simulink subsystem "TC_Target"  (R2021b)
settings: Solver=VariableStepAuto  StartTime=0.0  StopTime=10.0  RelTol=1e-3
undefined symbols (not defined in the file): afx_f, agx_f, BestSlipRate, gear_f, gear_r, Iwf, Load, mu_tire_F, Rwf, Rwr, SlipAngle
libraries: dspstat3 x2, simulink x2
settings Model: Creator=tsuyoshi  LastModifiedBy=tsuyoshi

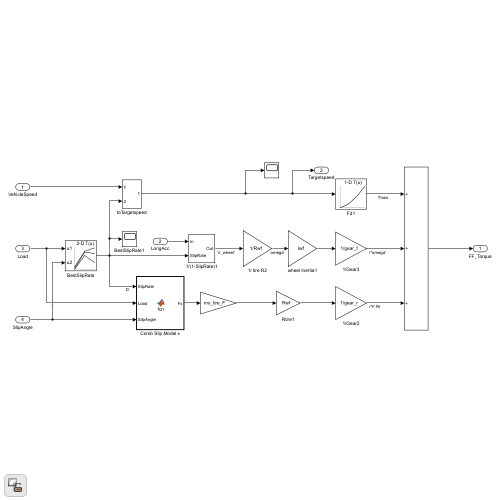
[thumbnail: Simulink's stored preview of the top-level diagram]
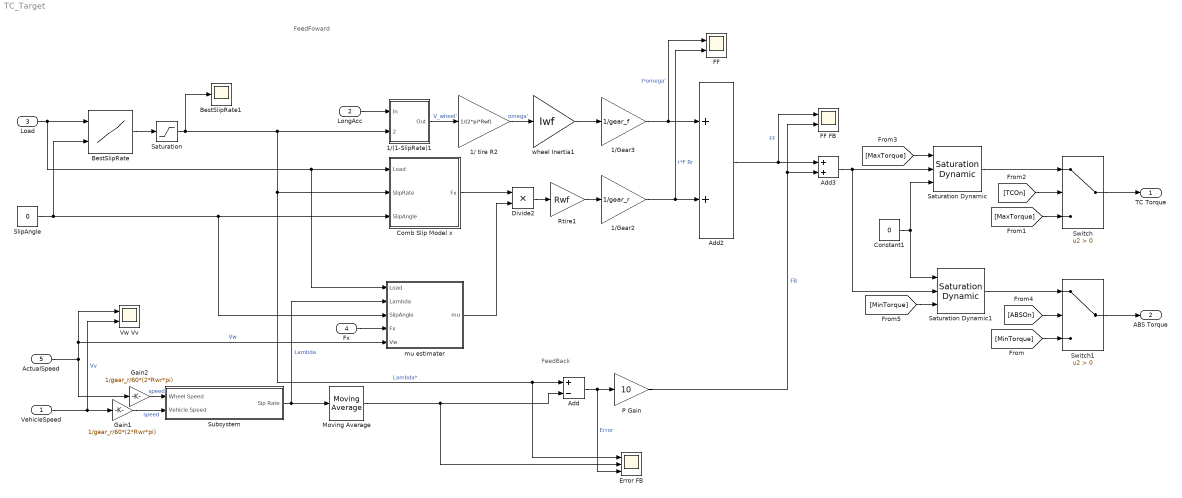
== system TC_Target ==
  note: FeedFoward
  note: FeedBack
  VehicleSpeed : Inport
  LongAcc : Inport  Port=2
  Load : Inport  Port=3
  Fx : Inport  Port=4
  ActualSpeed : Inport  Port=5
  1/ tire R2 : Gain  Gain=1/(2*pi*Rwf)
  1/(1-SlipRate)1 : Subsystem
  1/Gear2 : Gain  Gain=1/gear_r
  1/Gear3 : Gain  Gain=1/gear_f
  Add : Sum  Inputs=+-
  Add2 : Sum
  Add3 : Sum
  BestSlipRate : Lookup_n-D  BreakpointsForDimension1=Load  BreakpointsForDimension2=SlipAngle  Table=BestSlipRate  InternalRulePriority=Speed  RndMeth=Simplest  InputSameDT=on
      settings: InputPortMap=u0,u1
  BestSlipRate1 : Scope
  Comb Slip Model x : MATLAB Function  TreatAsAtomicUnit=on
  Constant1 : Constant  Value=0
  Divide2 : Product  Inputs=**
  Error FB : Scope  NumInputPorts=3
  FF : Scope  NumInputPorts=2
  FF FB : Scope  NumInputPorts=2
  Gain1 : Gain  Gain=1/gear_r/60*(2*Rwr*pi)
  Gain2 : Gain  Gain=1/gear_r/60*(2*Rwr*pi)
  Moving Average : dspstat3/Moving Average  Method=Sliding window  ForgettingFactorPort=off  SpecifyWindowLength=on  WindowLength=10  ForgettingFactor=0.9  SimulateUsing=Code generation
  P Gain : Gain  Gain=10
  Rtire1 : Gain  Gain=Rwf
  Saturation : Saturate  UpperLimit=0.3  LowerLimit=-0.3
  Saturation Dynamic : simulink/Discontinuities/Saturation Dynamic  OutMin=[]  OutMax=[]  OutDataTypeStr=Inherit: Same as second input  OutDataType=fixdt(1, 16)  OutScaling=2^-10  DoSatur=off
  Saturation Dynamic1 : simulink/Discontinuities/Saturation Dynamic  OutMin=[]  OutMax=[]  OutDataTypeStr=Inherit: Same as second input  OutDataType=fixdt(1, 16)  OutScaling=2^-10  DoSatur=off
  SlipAngle : Constant  Value=0
  Subsystem : Subsystem
  Switch : Switch  Criteria=u2 > Threshold
  Switch1 : Switch  Criteria=u2 > Threshold
  Vw Vv : Scope  NumInputPorts=2
  mu estimater : Subsystem
  wheel Inertia1 : Gain  Gain=Iwf
  TC Torque : Outport
  ABS Torque : Outport  Port=2
  wires:
  mu estimater/1(mu) -> Divide2/2
  Fx/1 -> mu estimater/4(Fx)
  Comb Slip Model x/1(Fx) -> Divide2/1
  Divide2/1 -> Rtire1/1
  Subsystem/1(Sip Rate) -> mu estimater/2(Lambda), Moving Average/1  "Lambda"
  Switch1/1 -> ABS Torque/1
  [MinTorque] -> Saturation Dynamic1/3
  Saturation Dynamic1/1 -> Switch1/1
  [ABSOn] -> Switch1/2
  [MinTorque] -> Switch1/3
  [MaxTorque] -> Saturation Dynamic/1
  Constant1/1 -> Saturation Dynamic/3, Saturation Dynamic1/1
  Switch/1 -> TC Torque/1
  Saturation Dynamic/1 -> Switch/1
  [TCOn] -> Switch/2
  Add3/1 -> Saturation Dynamic1/2, Saturation Dynamic/2
  [MaxTorque] -> Switch/3
  P Gain/1 -> Add3/2, FF FB/2  "FB"
  Add2/1 -> FF FB/1, Add3/1  "FF"
  Add/1 -> Error FB/3, P Gain/1  "Error"
  VehicleSpeed/1 -> Vw Vv/2, Gain1/1  "Vv"
  ActualSpeed/1 -> mu estimater/5(Vw), Vw Vv/1, Gain2/1  "Vw"
  BestSlipRate/1 -> Saturation/1
  SlipAngle/1 -> BestSlipRate/2, mu estimater/3(SlipAngle), Comb Slip Model x/3(SlipAngle)
  LongAcc/1 -> 1/(1-SlipRate)1/1(In)
  1/Gear3/1 -> FF/1, Add2/1  "I*omega'"
  1/ tire R2/1 -> wheel Inertia1/1  "omega'"
  Rtire1/1 -> 1/Gear2/1
  Load/1 -> mu estimater/1(Load), Comb Slip Model x/1(Load), BestSlipRate/1
  1/Gear2/1 -> FF/2, Add2/2  "r*F Rr"
  wheel Inertia1/1 -> 1/Gear3/1
  Saturation/1 -> 1/(1-SlipRate)1/2(SlipRate), Error FB/1, Add/1, Comb Slip Model x/2(SlipRate), BestSlipRate1/1  "Lambda*"
  1/(1-SlipRate)1/1(Out) -> 1/ tire R2/1  "V_wheel'"
  Gain1/1 -> Subsystem/2(Vehicle Speed)  "speed"
  Gain2/1 -> Subsystem/1(Wheel Speed)  "speed"
  Moving Average/1 -> Add/2, Error FB/2

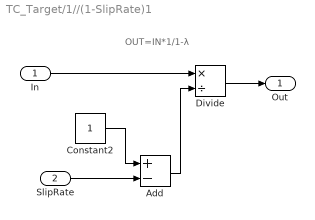
== system TC_Target/1//(1-SlipRate)1 ==
  note: OUT=IN*1/1-λ
  In : Inport
  SlipRate : Inport  Port=2
  Add : Sum  Inputs=+-
  Constant2 : Constant
  Divide : Product  Inputs=*/
  Out : Outport
  wires:
  Constant2/1 -> Add/1
  Add/1 -> Divide/2
  SlipRate/1 -> Add/2
  Divide/1 -> Out/1
  In/1 -> Divide/1

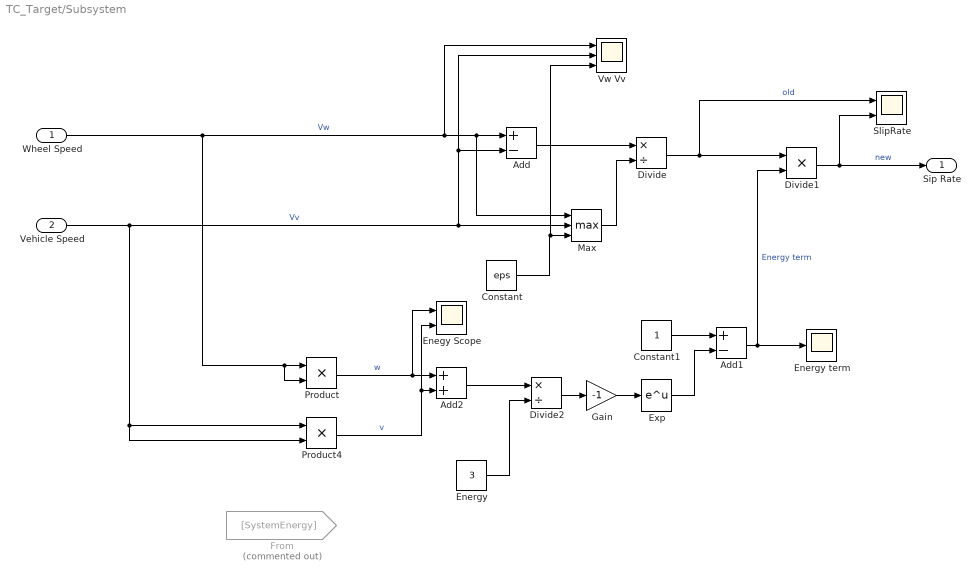
== system TC_Target/Subsystem ==
  Wheel Speed : Inport
  Vehicle Speed : Inport  Port=2
  Add : Sum  Inputs=+-
  Add1 : Sum  Inputs=+-
  Add2 : Sum
  Constant : Constant  Value=eps
  Constant1 : Constant
  Divide : Product  Inputs=*/
  Divide1 : Product  Inputs=**
  Divide2 : Product  Inputs=*/
  Enegy Scope : Scope  NumInputPorts=2
  Energy : Constant  Value=3
  Energy term : Scope
  Exp : Math  SaturateOnIntegerOverflow=on
  From : From  Commented=on  GotoTag=SystemEnergy  TagVisibility=global
  Gain : Gain  Gain=-1
  Max : MinMax  Function=max  Inputs=3
  Product : Product
  Product4 : Product
  SlipRate : Scope  NumInputPorts=2
  Vw Vv : Scope  NumInputPorts=3
  Sip Rate : Outport  VectorParamsAs1DForOutWhenUnconnected=off
  wires:
  Divide2/1 -> Gain/1
  Constant/1 -> Max/3, Vw Vv/3
  Gain/1 -> Exp/1
  Max/1 -> Divide/2
  Divide/1 -> Divide1/1, SlipRate/1  "old"
  Wheel Speed/1 -> Max/1, Add/1, Vw Vv/1, Product/2, Product/1  "Vw"
  Divide1/1 -> SlipRate/2, Sip Rate/1  "new"
  Product4/1 -> Enegy Scope/2, Add2/2  "v"
  Exp/1 -> Add1/2
  Energy/1 -> Divide2/2
  Vehicle Speed/1 -> Product4/1, Product4/2, Vw Vv/2, Add/2, Max/2  "Vv"
  Add1/1 -> Divide1/2, Energy term/1  "Energy term"
  Add/1 -> Divide/1
  Constant1/1 -> Add1/1
  Add2/1 -> Divide2/1
  Product/1 -> Add2/1, Enegy Scope/1  "w"

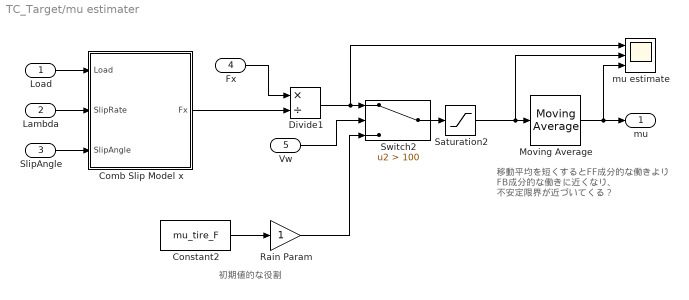
== system TC_Target/mu estimater ==
  note: 初期値的な役割
  note: 移動平均を短くするとFF成分的な働きより
      | FB成分的な働きに近くなり、
      | 不安定限界が近づいてくる？
  Load : Inport
  Lambda : Inport  Port=2
  SlipAngle : Inport  Port=3
  Fx : Inport  Port=4
  Vw : Inport  Port=5
  Comb Slip Model x : MATLAB Function  TreatAsAtomicUnit=on
  Constant2 : Constant  Value=mu_tire_F
  Divide1 : Product  Inputs=*/
  Moving Average : dspstat3/Moving Average  Method=Sliding window  ForgettingFactorPort=off  SpecifyWindowLength=on  WindowLength=100  ForgettingFactor=0.9  SimulateUsing=Code generation
  Rain Param : Gain
  Saturation2 : Saturate  UpperLimit=0.7  LowerLimit=0.1
  Switch2 : Switch  Criteria=u2 > Threshold  Threshold=100
  mu estimate : Scope  NumInputPorts=3
  mu : Outport
  wires:
  Rain Param/1 -> Switch2/3
  Constant2/1 -> Rain Param/1
  Saturation2/1 -> mu estimate/2, Moving Average/1
  Fx/1 -> Divide1/1
  Moving Average/1 -> mu estimate/3, mu/1
  Divide1/1 -> mu estimate/1, Switch2/1
  Vw/1 -> Switch2/2
  Switch2/1 -> Saturation2/1
  Comb Slip Model x/1(Fx) -> Divide1/2
  Load/1 -> Comb Slip Model x/1(Load)
  Lambda/1 -> Comb Slip Model x/2(SlipRate)
  SlipAngle/1 -> Comb Slip Model x/3(SlipAngle)

== matlab function TC_Target/Comb Slip Model x ==
  data: Load input; SlipRate input; Fx output; SlipAngle input; agx_f parameter; afx_f parameter
function Fx = fcn(Load, SlipRate, SlipAngle, agx_f, afx_f)
    if Load==0
        Fx=0;
    else
        C = agx_f(1);
        D = fcnPureFx(Load, SlipRate, afx_f);
        E = Load*agx_f(4) + agx_f(5);
        B = agx_f(2)*sin(2*atan(Load/agx_f(3)))/(D*C);
        Fx = D*cos(C*atan(B*SlipAngle-E*(B*SlipAngle-atan(B*SlipAngle))));
    end
end

function PureFx = fcnPureFx(Load, SlipRate, afx_f)
    C = afx_f(1);
    D = (Load*afx_f(2) + afx_f(3))*Load;
    E = Load*afx_f(6) + afx_f(7);
    B = afx_f(4)*sin(2*atan(Load/afx_f(5)))/(D*C);
    PureFx = D*sin(C*atan(B*SlipRate-E*(B*SlipRate-atan(B*SlipRate))));
end

== matlab function TC_Target/mu estimater/Comb Slip Model x ==
  data: Load input; SlipRate input; Fx output; SlipAngle input; agx_f parameter; afx_f parameter
function Fx = fcn(Load, SlipRate, SlipAngle, agx_f, afx_f)
    if Load==0
        Fx=0;
    else
        C = agx_f(1);
        D = fcnPureFx(Load, SlipRate, afx_f);
        E = Load*agx_f(4) + agx_f(5);
        B = agx_f(2)*sin(2*atan(Load/agx_f(3)))/(D*C);
        Fx = D*cos(C*atan(B*SlipAngle-E*(B*SlipAngle-atan(B*SlipAngle))));
    end
end

function PureFx = fcnPureFx(Load, SlipRate, afx_f)
    C = afx_f(1);
    D = (Load*afx_f(2) + afx_f(3))*Load;
    E = Load*afx_f(6) + afx_f(7);
    B = afx_f(4)*sin(2*atan(Load/afx_f(5)))/(D*C);
    PureFx = D*sin(C*atan(B*SlipRate-E*(B*SlipRate-atan(B*SlipRate))));
end
